simulink model "pll_5"  (Simulink 3.00)
settings: Solver=ode45  SolverMode=SingleTasking  StartTime=0.0  StopTime=0.5  RelTol=1e-3  AbsTol=1e-6
values from neighbouring files (symbols this model uses):
  f0 = 500    [chirp_1.m]    (also in costas1f.m = pf0; op_freq.m = 15; pll_5f.m = f01)
  kvco = pkvco    [costas1f.m]    (also in pll_5f.m = kvco1)
  ph_fehler = p_ph_fehler    [costas1f.m]    (also in pll_5f.m = ph_fehler1)
  tau = ptau    [costas1f.m]    (also in op_freq.m = 0.0106103295395; pll_5f.m = tau1)
settings Model: Refine=3

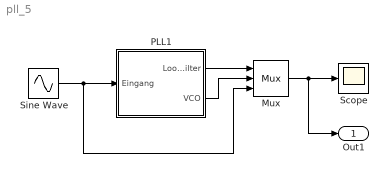
== system pll_5 ==
  Mux : Mux  Inputs=3
      settings: DisplayOption=none
  PLL1 : Subsystem
  Scope : Scope
      settings: TickLabels=on  TimeRange=auto  YMin=-5  YMax=5  SaveToWorkspace=off  SaveName=ScopeData  DataFormat=Matrix
  Sine Wave : Sin  Amplitude=1  Frequency=2*pi*f0  Phase=0  SampleTime=0
  Out1 : Outport  Port=1
  wires:
  PLL1/1(Loop-Filter) -> Mux/1
  PLL1/2(" VCO") -> Mux/2
  Sine Wave/1 -> PLL1/1(Eingang), Mux/3
  Mux/1 -> Scope/1, Out1/1

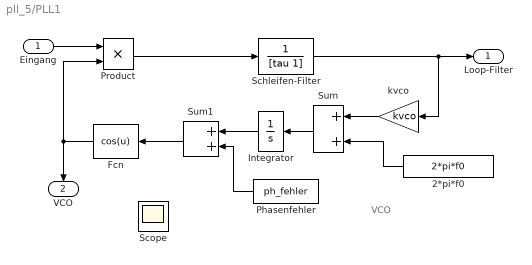
== system pll_5/PLL1 ==
  note: VCO
  Eingang : Inport  Port=1  PortWidth=-1  SampleTime=-1  DataType=auto
      settings: SignalType=auto
  2*pi*f0 : Constant  Orientation=left  Value=2*pi*f0
  Fcn : Fcn  Orientation=left  Expr=cos(u)
  Integrator : Integrator  Orientation=left  ExternalReset=none  InitialConditionSource=internal  InitialCondition=0  LimitOutput=off  UpperSaturationLimit=inf  LowerSaturationLimit=-inf  ShowSaturationPort=off  ShowStatePort=off  AbsoluteTolerance=auto
  Phasenfehler : Constant  Orientation=left  Value=ph_fehler
  Product : Product  Inputs=2  SaturateOnIntegerOverflow=on
  Schleifen-Filter : TransferFcn  Numerator=[1]  Denominator=[tau 1]
  Scope : Scope
      settings: Floating=on  TickLabels=on  TimeRange=0.1  YMin=-5  YMax=5  SaveToWorkspace=off  SaveName=ScopeData  DataFormat=Matrix
  Sum : Sum  Orientation=left  Inputs=++  SaturateOnIntegerOverflow=on
  Sum1 : Sum  Orientation=left  Inputs=++  SaturateOnIntegerOverflow=on
  kvco : Gain  Orientation=left  Gain=kvco  SaturateOnIntegerOverflow=on
  Loop-Filter : Outport  Port=1  InitialOutput=0
  " VCO" : Outport  Orientation=down  Port=2  InitialOutput=0
  wires:
  Fcn/1 -> Product/2, " VCO"/1
  Eingang/1 -> Product/1
  Sum1/1 -> Fcn/1
  Product/1 -> Schleifen-Filter/1
  Sum/1 -> Integrator/1
  2*pi*f0/1 -> Sum/2
  kvco/1 -> Sum/1
  Schleifen-Filter/1 -> kvco/1, Loop-Filter/1
  Phasenfehler/1 -> Sum1/2
  Integrator/1 -> Sum1/1
